simulink model "nnex"  (Simulink 3.00)
settings: Solver=ode4  StartTime=0.0  StopTime=80.0  FixedStep=0.01  RelTol=1e-3
values from neighbouring files (symbols this model uses):
  a = [0 0 0 0 -1.84243174515 0 -13.0175486382 0 -0.783906463276 0 0 0 ... (81 elements, 9x9)]    [abcdkkf.mat]
  b = [0 0 0 0.0409816056965 -1.1184911635 -0.696996430025 -7.90261427727 -0.243253277751 -0.475887299716 0 0 0 ... (72 elements, 9x8)]    [abcdkkf.mat]
  K = [0.205046990931 0.178802882473 0.205046973039 0.231291081498 0.205047227102 0.208989425276 0.205046736869 0.201104538695 0.029790172361 1.88182262784e-07 -0.0297901447303 -1.60551558311e-07 ... (72 elements, 8x9)]    [abcdkkf.mat]
  Kf = [-0.016083954489 -0.0112761944666 -0.0160839192866 -0.020891679309 -0.0160839730143 0.0019082921562 -0.0160839007613 -0.0340761659318 -0.0453569952473 -2.86516704076e-07 0.0453569531782 2.44447604365e-07 ... (24 elements, 8x3)]    [abcdkkf.mat]
undefined symbols (not defined in the file or in its folder): h, Kd, Kp, omega, zeta
libraries: smxl x11, simulink3 x6, neural x2
settings Model: LastModifiedBy=giampiero

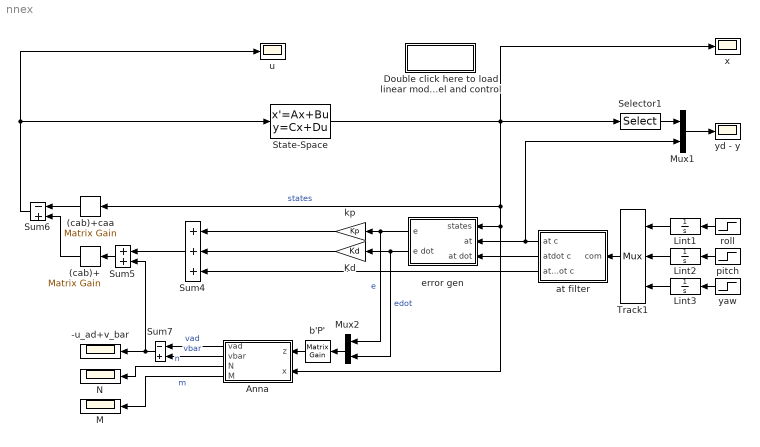
== system nnex ==
  (cab)+ : simulink3/Math/Matrix Gain  Orientation=left  K=Kf
  (cab)+caa : simulink3/Math/Matrix Gain  Orientation=left  K=K
  -u_ad+v_bar : Scope
      settings: TickLabels=off  TimeRange=40  YMin=-250  YMax=50  SaveName=u_nn  DataFormat=Matrix  MaxRows=40000
  Anna : Subsystem  Orientation=left  mask(Adaptive Neural Network){s=[     3    9      6     1       0         0        0], g=[0.1         40     0   40 40           0.01]}
      mask prompts: s "[nno nni nnh act rndN rndM bias]"; g "[Kv   Z_bar   Kz    G   F   lambda]"
      mask help: Continuous Time Adaptive Multilayer MIMO Neural Network.
      mask init:
      | nno=s(1); nni=s(2); nnh=s(3); a=s(4); rndN=s(5);rndM=s(6);
      | bias=s(7); Kv=g(1); Z_bar=g(2);Kz=g(3);G=g(4);F=g(5);lam=g(6);
      mask Help:
      | <html xmlns:o="urn:schemas-microsoft-com:office:office"
      | xmlns:w="urn:schemas-microsoft-com:office:word"
      | xmlns="http://www.w3.org/TR/REC-html40">
      | 
      | <head>
      | <meta http-equiv=Content-Type content="text/html; charset=windows-1252">
      | <meta name=ProgId content=Word.Document>
      | <meta name=Generator content="Microsoft Word 9">
      | <meta name=Originator content="Microsoft Word 9">
      | <link rel=File-List href="./help_files/filelist.xml">
      | <title>Notation and adaptation algorithm are taken from the paper:</title>
      | <!--[if gte mso 9]><xml>
      |  <o:DocumentProperties>
      |   <o:Author>Control Lab</o:Author>
      |   <o:LastAuthor>giampiero</o:LastAuthor>
      |   <o:Revision>14</o:Revision>
      |   <o:TotalTime>134</o:TotalTime>
      |   <o:Created>1999-07-30T18:31:00Z</o:Created>
      |   <o:LastSaved>2000-05-30T23:27:00Z</o:LastSaved>
      |   <o:Pages>1</o:Pages>
      |   <o:Words>234</o:Words>
      |   <o:Characters>1339</o:Characters>
      |   <o:Company>GA TECH</o:Company>
      |   <o:Lines>11</o:Lines>
      |   <o:Paragraphs>2</o:Paragraphs>
      |   <o:CharactersWithSpaces>1644</o:CharactersWithSpaces>
      |   <o:Version>9.2720</o:Version>
      |  </o:DocumentProperties>
      | </xml><![endif]-->
      | <style>
      | <!--
      |  /* Style Definitions */
      | p.MsoNormal, li.MsoNormal, div.MsoNormal
      | 	{mso-style-parent:"";
      | 	margin:0in;
      | 	margin-bottom:.0001pt;
      | 	mso-pagination:widow-orphan;
      | 	font-size:12.0pt;
      | 	font-family:"Times New Roman";
      | 	mso-fareast-font-family:"Times New Roman";}
      | p.MsoBodyText, li.MsoBodyText, div.MsoBodyText
      | 	{margin-top:0in;
      | 	margin-right:3.35in;
      | 	margin-bottom:0in;
      | 	margin-left:0in;
      | 	margin-bottom:.0001pt;
      | 	mso-pagination:widow-orphan;
      | 	font-size:12.0pt;
      | 	font-family:"Times New Roman";
      | 	mso-fareast-font-family:"Times New Roman";}
      | p.MsoBodyText2, li.MsoBodyText2, div.MsoBodyText2
      | 	{margin-top:0in;
      | 	margin-right:2.35in;
      | 	margin-bottom:0in;
      | 	margin-left:0in;
      | 	margin-bottom:.0001pt;
      | 	mso-pagination:widow-orphan;
      | 	font-size:12.0pt;
      | 	font-family:"Times New Roman";
      | 	mso-fareast-font-family:"Times New Roman";}
      | @page Section1
      | 	{size:8.5in 11.0in;
      | 	margin:1.0in 1.25in 1.0in 1.25in;
      | 	mso-header-margin:.5in;
      | 	mso-footer-margin:.5in;
      | 	mso-paper-source:0;}
      | div.Section1
      | 	{page:Section1;}
      |  /* List Definitions */
      | @list l0
      | 	{mso-list-id:387336931;
      | 	mso-list-type:hybrid;
      | 	mso-list-template-ids:1661509918 67698705 67698713 67698715 67698703 67698713 67698715 67698703 67698713 67698715;}
      | @list l0:level1
      | 	{mso-level-text:"%1\)";
      | 	mso-level-tab-stop:.5in;
      | 	mso-level-number-position:left;
      | 	text-indent:-.25in;}
      | @list l1
      | 	{mso-list-id:1390807613;
      | 	mso-list-type:hybrid;
      | 	mso-list-template-ids:210782786 67698705 67698713 67698715 67698703 67698713 67698715 67698703 67698713 67698715;}
      | @list l1:level1
      | 	{mso-level-text:"%1\)";
      | 	mso-level-tab-stop:.5in;
      | 	mso-level-number-position:left;
      | 	text-indent:-.25in;}
      | @list l2
      | 	{mso-list-id:1468430361;
      | 	mso-list-type:hybrid;
      | 	mso-list-template-ids:-783395272 67698705 67698713 67698715 67698703 67698713 67698715 67698703 67698713 67698715;}
      | @list l2:level1
      | 	{mso-level-text:"%1\)";
      | 	mso-level-tab-stop:.5in;
      | 	mso-level-number-position:left;
      | 	text-indent:-.25in;}
      | @list l3
      | 	{mso-list-id:2055232913;
      | 	mso-list-type:hybrid;
      | 	mso-list-template-ids:-1797358054 67698705 67698713 67698715 67698703 67698713 67698715 67698703 67698713 67698715;}
      | @list l3:level1
      | 	{mso-level-text:"%1\)";
      | 	mso-level-tab-stop:.5in;
      | 	mso-level-number-position:left;
      | 	text-indent:-.25in;}
      | ol
      | 	{margin-bottom:0in;}
      | ul
      | 	{margin-bottom:0in;}
      | -->
      | </style>
      | </head>
      | 
      | <body lang=EN-US style='tab-interval:.5in'>
      | 
      | <div class=Section1>
      | 
      | <p class=MsoBodyText2 style='margin-right:-1.8pt'>The block implements a
      | continuous time adaptive multilayer MIMO sigmoidal neural network, this is a
      | simulink based version that uses the Transposition and Multiplication blocks from the Smxl Library, therefore you must have that library in your Matlab path in order to use this block.</p>
      | 
      | <p class=MsoNormal style='margin-right:-1.8pt'><![if !supportEmptyParas]>&nbsp;<![endif]><o:p></o:p></p>
      | 
      | <p class=MsoNormal style='margin-right:-1.8pt'>Notation and adaptation
      | algorithm are taken from the paper:</p>
      | 
      | <p class=MsoBodyText style='margin-right:-1.8pt'>Neural Network Based Adaptive
      | Control of a Thrust Vectored Fan, Nardi, Rysdik, Calise, AIAA 1999-3996, where
      | the used neural network has the equations shown below:</p>
      | 
      | <p class=MsoBodyText style='margin-right:-1.8pt'><![if !supportEmptyParas]>&nbsp;<![endif]><o:p></o:p></p>
      | 
      | <p class=MsoBodyText style='margin-right:-1.8pt;tab-stops:27.0pt'>N<sub>dot<span
      | style='mso-tab-count:1'>    </span></sub>= -G[x<sub>bar</sub><span
      | style='font-family:Symbol;mso-ascii-font-family:"Times New Roman";mso-hansi-font-family:
      | "Times New Roman";mso-char-type:symbol;mso-symbol-font-family:Symbol'><span
      | style='mso-char-type:symbol;mso-symbol-font-family:Symbol'>z</span></span>M<sup>T</sup><span
      | style='font-family:Symbol;mso-ascii-font-family:"Times New Roman";mso-hansi-font-family:
      | "Times New Roman";mso-char-type:symbol;mso-symbol-font-family:Symbol'><span
      | style='mso-char-type:symbol;mso-symbol-font-family:Symbol'>s</span></span>’(N<sup>T</sup>x<sub>bar</sub>)
      | + <span style='font-family:Symbol;mso-ascii-font-family:"Times New Roman";
      | mso-hansi-font-family:"Times New Roman";mso-char-type:symbol;mso-symbol-font-family:
      | Symbol'><span style='mso-char-type:symbol;mso-symbol-font-family:Symbol'>l</span></span><span
      | style='font-family:Symbol;mso-ascii-font-family:"Times New Roman";mso-hansi-font-family:
      | "Times New Roman";mso-char-type:symbol;mso-symbol-font-family:Symbol'><span
      | style='mso-char-type:symbol;mso-symbol-font-family:Symbol'>ï</span></span><span
      | style='font-family:Symbol;mso-ascii-font-family:"Times New Roman";mso-hansi-font-family:
      | "Times New Roman";mso-char-type:symbol;mso-symbol-font-family:Symbol'><span
      | style='mso-char-type:symbol;mso-symbol-font-family:Symbol'>z</span></span><span
      | style='font-family:Symbol;mso-ascii-font-family:"Times New Roman";mso-hansi-font-family:
      | "Times New Roman";mso-char-type:symbol;mso-symbol-font-family:Symbol'><span
      | style='mso-char-type:symbol;mso-symbol-font-family:Symbol'>ï</span></span>N]</p>
      | 
      | <p class=MsoBodyText style='margin-right:-1.8pt;tab-stops:27.0pt'>N<sub>dot<span
      | style='mso-tab-count:1'>    </span></sub>= -F[(<span style='font-family:Symbol;
      | mso-ascii-font-family:"Times New Roman";mso-hansi-font-family:"Times New Roman";
      | mso-char-type:symbol;mso-symbol-font-family:Symbol'><span style='mso-char-type:
      | symbol;mso-symbol-font-family:Symbol'>s</span></span>(N<sup>T</sup>x<sub>bar</sub>)-<span
      | style='font-family:Symbol;mso-ascii-font-family:"Times New Roman";mso-hansi-font-family:
      | "Times New Roman";mso-char-type:symbol;mso-symbol-font-family:Symbol'><span
      | style='mso-char-type:symbol;mso-symbol-font-family:Symbol'>s</span></span>’(N<sup>T</sup>x<sub>bar</sub>)N<sup>T</sup>x<sub>bar</sub>)<span
      | style='font-family:Symbol;mso-ascii-font-family:"Times New Roman";mso-hansi-font-family:
      | "Times New Roman";mso-char-type:symbol;mso-symbol-font-family:Symbol'><span
      | style='mso-char-type:symbol;mso-symbol-font-family:Symbol'>z</span></span> + <span
      | style='font-family:Symbol;mso-ascii-font-family:"Times New Roman";mso-hansi-font-family:
      | "Times New Roman";mso-char-type:symbol;mso-symbol-font-family:Symbol'><span
      | style='mso-char-type:symbol;mso-symbol-font-family:Symbol'>l</span></span><span
      | style='font-family:Symbol;mso-ascii-font-family:"Times New Roman";mso-hansi-font-family:
      | "Times New Roman";mso-char-type:symbol;mso-symbol-font-family:Symbol'><span
      | style='mso-char-type:symbol;mso-symbol-font-family:Symbol'>ï</span></span><span
      | style='font-family:Symbol;mso-ascii-font-family:"Times New Roman";mso-hansi-font-family:
      | "Times New Roman";mso-char-type:symbol;mso-symbol-font-family:Symbol'><span
      | style='mso-char-type:symbol;mso-symbol-font-family:Symbol'>z</span></span><span
      | style='font-family:Symbol;mso-ascii-font-family:"Times New Roman";mso-hansi-font-family:
      | "Times New Roman";mso-char-type:symbol;mso-symbol-font-family:Symbol'><span
      | style='mso-char-type:symbol;mso-symbol-font-family:Symbol'>ï</span></span>M]</p>
      | 
      | <p class=MsoBodyText style='margin-right:-1.8pt;tab-stops:27.0pt'>v<sub>ad<span
      | style='mso-tab-count:1'>       </span></sub>= <span style="mso-spacerun:
      | yes"> </span>M<sup>T</sup><span style='font-family:Symbol;mso-ascii-font-family:
      | "Times New Roman";mso-hansi-font-family:"Times New Roman";mso-char-type:symbol;
      | mso-symbol-font-family:Symbol'><span style='mso-char-type:symbol;mso-symbol-font-family:
      | Symbol'>s</span></span>(N<sup>T</sup>x<sub>bar</sub>)</p>
      | 
      | <p class=MsoBodyText style='margin-right:-1.8pt;tab-stops:27.0pt'>v<sub>bar<span
      | style='mso-tab-count:1'>      </span></sub>= <span style="mso-spacerun:
      | yes"> </span>K<sub>v</sub> (<span style='font-family:Symbol;mso-ascii-font-family:
      | "Times New Roman";mso-hansi-font-family:"Times New Roman";mso-char-type:symbol;
      | mso-symbol-font-family:Symbol'><span style='mso-char-type:symbol;mso-symbol-font-family:
      | Symbol'>ï</span></span>Z<span style='font-family:Symbol;mso-ascii-font-family:
      | "Times New Roman";mso-hansi-font-family:"Times New Roman";mso-char-type:symbol;
      | mso-symbol-font-family:Symbol'><span style='mso-char-type:symbol;mso-symbol-font-family:
      | Symbol'>ï</span></span><sub>F</sub> + Z<sub>bar</sub>)<span style='font-family:
      | Symbol;mso-ascii-font-family:"Times New Roman";mso-hansi-font-family:"Times New Roman";
      | mso-char-type:symbol;mso-symbol-font-family:Symbol'><span style='mso-char-type:
      | symbol;mso-symbol-font-family:Symbol'>z</span></span><sup>T</sup> + K<sub>z</sub><span
      | style='font-family:Symbol;mso-ascii-font-family:"Times New Roman";mso-hansi-font-family:
      | "Times New Roman";mso-char-type:symbol;mso-symbol-font-family:Symbol'><span
      | style='mso-char-type:symbol;mso-symbol-font-family:Symbol'>z</span></span><sup>T</sup></p>
      | 
      | <p class=MsoBodyText style='margin-right:-1.8pt'><![if !supportEmptyParas]>&nbsp;<![endif]><o:p></o:p></p>
      | 
      | <p class=MsoNormal style='margin-right:-1.8pt'>The <u>Inputs</u> are:</p>
      | 
      | <p class=MsoNormal style='margin-top:0in;margin-right:-1.8pt;margin-bottom:
      | 0in;margin-left:.5in;margin-bottom:.0001pt;text-indent:-.25in;mso-list:l2 level1 lfo2;
      | tab-stops:list .5in'><![if !supportLists]>1)<span style='font:7.0pt "Times New Roman"'>&nbsp;&nbsp;&nbsp;&nbsp;&nbsp;
      | </span><![endif]>error vector <span style='font-family:Symbol;mso-ascii-font-family:
      | "Times New Roman";mso-hansi-font-family:"Times New Roman";mso-char-type:symbol;
      | mso-symbol-font-family:Symbol'><span style='mso-char-type:symbol;mso-symbol-font-family:
      | Symbol'>z</span></span> (<span style='font-family:Symbol;mso-ascii-font-family:
      | "Times New Roman";mso-hansi-font-family:"Times New Roman";mso-char-type:symbol;
      | mso-symbol-font-family:Symbol'><span style='mso-char-type:symbol;mso-symbol-font-family:
      | Symbol'>z</span></span>=ePb).</p>
      | 
      | <p class=MsoNormal style='margin-top:0in;margin-right:-1.8pt;margin-bottom:
      | 0in;margin-left:.5in;margin-bottom:.0001pt;text-indent:-.25in;mso-list:l2 level1 lfo2;
      | tab-stops:list .5in'><![if !supportLists]>2)<span style='font:7.0pt "Times New Roman"'>&nbsp;&nbsp;&nbsp;&nbsp;&nbsp;
      | </span><![endif]>net input vector x<sub>bar</sub> (x<sub>bar</sub>=[x,u]).</p>
      | 
      | <p class=MsoNormal style='margin-right:-1.8pt'><![if !supportEmptyParas]>&nbsp;<![endif]><o:p></o:p></p>
      | 
      | <p class=MsoNormal style='margin-right:-1.8pt'>The <u>States</u> are all N and
      | M entries.</p>
      | 
      | <p class=MsoNormal style='margin-right:-1.8pt'><![if !supportEmptyParas]>&nbsp;<![endif]><o:p></o:p></p>
      | 
      | <p class=MsoNormal style='margin-right:-1.8pt;text-align:justify'>The <u>Outputs</u>
      | are:</p>
      | 
      | <p class=MsoNormal style='margin-top:0in;margin-right:-1.8pt;margin-bottom:
      | 0in;margin-left:.5in;margin-bottom:.0001pt;text-indent:-.25in;mso-list:l1 level1 lfo4;
      | tab-stops:list .5in'><![if !supportLists]>1)<span style='font:7.0pt "Times New Roman"'>&nbsp;&nbsp;&nbsp;&nbsp;&nbsp;
      | </span><![endif]>v<sub>ad</sub> (adaptive contribution).</p>
      | 
      | <p class=MsoNormal style='margin-top:0in;margin-right:-1.8pt;margin-bottom:
      | 0in;margin-left:.5in;margin-bottom:.0001pt;text-indent:-.25in;mso-list:l1 level1 lfo4;
      | tab-stops:list .5in'><![if !supportLists]>2)<span style='font:7.0pt "Times New Roman"'>&nbsp;&nbsp;&nbsp;&nbsp;&nbsp;
      | </span><![endif]>v<sub>bar</sub> ( robustifying contribution).</p>
      | 
      | <p class=MsoNormal style='margin-top:0in;margin-right:-1.8pt;margin-bottom:
      | 0in;margin-left:.5in;margin-bottom:.0001pt;text-indent:-.25in;mso-list:l1 level1 lfo4;
      | tab-stops:list .5in'><![if !supportLists]>3)<span style='font:7.0pt "Times New Roman"'>&nbsp;&nbsp;&nbsp;&nbsp;&nbsp;
      | </span><![endif]>N entries taken columnwise.</p>
      | 
      | <p class=MsoNormal style='margin-top:0in;margin-right:-1.8pt;margin-bottom:
      | 0in;margin-left:.5in;margin-bottom:.0001pt;text-indent:-.25in;mso-list:l1 level1 lfo4;
      | tab-stops:list .5in'><![if !supportLists]>4)<span style='font:7.0pt "Times New Roman"'>&nbsp;&nbsp;&nbsp;&nbsp;&nbsp;
      | </span><![endif]>M entries taken columnwise.</p>
      | 
      | <p class=MsoNormal style='margin-right:-1.8pt'><![if !supportEmptyParas]>&nbsp;<![endif]><o:p></o:p></p>
      | 
      | <p class=MsoNormal style='margin-right:-1.8pt'>The <u>first</u> parameter must
      | be a vector containing:</p>
      | 
      | <p class=MsoNormal style='margin-top:0in;margin-right:-1.8pt;margin-bottom:
      | 0in;margin-left:.5in;margin-bottom:.0001pt;text-indent:-.25in;mso-list:l0 level1 lfo6;
      | tab-stops:list .5in'><![if !supportLists]>1)<span style='font:7.0pt "Times New Roman"'>&nbsp;&nbsp;&nbsp;&nbsp;&nbsp;
      | </span><![endif]>nno = number of network output = size of the error.</p>
      | 
      | <p class=MsoNormal style='margin-top:0in;margin-right:-1.8pt;margin-bottom:
      | 0in;margin-left:.5in;margin-bottom:.0001pt;text-indent:-.25in;mso-list:l0 level1 lfo6;
      | tab-stops:list .5in'><![if !supportLists]>2)<span style='font:7.0pt "Times New Roman"'>&nbsp;&nbsp;&nbsp;&nbsp;&nbsp;
      | </span><![endif]>nni = number of network inputs = plant states.</p>
      | 
      | <p class=MsoNormal style='margin-top:0in;margin-right:-1.8pt;margin-bottom:
      | 0in;margin-left:.5in;margin-bottom:.0001pt;text-indent:-.25in;mso-list:l0 level1 lfo6;
      | tab-stops:list .5in'><![if !supportLists]>3)<span style='font:7.0pt "Times New Roman"'>&nbsp;&nbsp;&nbsp;&nbsp;&nbsp;
      | </span><![endif]>nnh = number of hidden layer neurons.</p>
      | 
      | <p class=MsoNormal style='margin-top:0in;margin-right:-1.8pt;margin-bottom:
      | 0in;margin-left:.5in;margin-bottom:.0001pt;text-indent:-.25in;mso-list:l0 level1 lfo6;
      | tab-stops:list .5in'><![if !supportLists]>4)<span style='font:7.0pt "Times New Roman"'>&nbsp;&nbsp;&nbsp;&nbsp;&nbsp;
      | </span><![endif]>act = sigmoid activation potential.</p>
      | 
      | <p class=MsoNormal style='margin-top:0in;margin-right:-1.8pt;margin-bottom:
      | 0in;margin-left:.5in;margin-bottom:.0001pt;text-indent:-.25in;mso-list:l0 level1 lfo6;
      | tab-stops:list .5in'><![if !supportLists]>5)<span style='font:7.0pt "Times New Roman"'>&nbsp;&nbsp;&nbsp;&nbsp;&nbsp;
      | </span><![endif]>rndN = multiplies random initial weights N.</p>
      | 
      | <p class=MsoNormal style='margin-top:0in;margin-right:-1.8pt;margin-bottom:
      | 0in;margin-left:.5in;margin-bottom:.0001pt;text-indent:-.25in;mso-list:l0 level1 lfo6;
      | tab-stops:list .5in'><![if !supportLists]>6)<span style='font:7.0pt "Times New Roman"'>&nbsp;&nbsp;&nbsp;&nbsp;&nbsp;
      | </span><![endif]>rndM = multiplies random initial weights M.</p>
      | 
      | <p class=MsoNormal style='margin-top:0in;margin-right:-1.8pt;margin-bottom:
      | 0in;margin-left:.5in;margin-bottom:.0001pt;text-indent:-.25in;mso-list:l0 level1 lfo6;
      | tab-stops:list .5in'><![if !supportLists]>7)<span style='font:7.0pt "Times New Roman"'>&nbsp;&nbsp;&nbsp;&nbsp;&nbsp;
      | </span><![endif]>bias = put 1 if you want it, 0 otherwise.</p>
      | 
      | <p class=MsoNormal style='margin-right:-1.8pt'><![if !supportEmptyParas]>&nbsp;<![endif]><o:p></o:p></p>
      | 
      | <p class=MsoBodyText style='margin-right:-1.8pt'>The <u>second</u> parameter
      | must be a vector containing:</p>
      | 
      | <p class=MsoNormal style='margin-top:0in;margin-right:-1.8pt;margin-bottom:
      | 0in;margin-left:.5in;margin-bottom:.0001pt;text-indent:-.25in;mso-list:l3 level1 lfo8;
      | tab-stops:list .5in'><![if !supportLists]>1)<span style='font:7.0pt "Times New Roman"'>&nbsp;&nbsp;&nbsp;&nbsp;&nbsp;
      | </span><![endif]>K<sub>v</sub> = multiplies first term of v<sub>bar</sub>.</p>
      | 
      | <p class=MsoNormal style='margin-top:0in;margin-right:-1.8pt;margin-bottom:
      | 0in;margin-left:.5in;margin-bottom:.0001pt;text-indent:-.25in;mso-list:l3 level1 lfo8;
      | tab-stops:list .5in'><![if !supportLists]>2)<span style='font:7.0pt "Times New Roman"'>&nbsp;&nbsp;&nbsp;&nbsp;&nbsp;
      | </span><![endif]>Z<sub>bar</sub> = maximum expected <span style='font-family:
      | Symbol;mso-ascii-font-family:"Times New Roman";mso-hansi-font-family:"Times New Roman";
      | mso-char-type:symbol;mso-symbol-font-family:Symbol'><span style='mso-char-type:
      | symbol;mso-symbol-font-family:Symbol'>ï</span></span>Z<span style='font-family:
      | Symbol;mso-ascii-font-family:"Times New Roman";mso-hansi-font-family:"Times New Roman";
      | mso-char-type:symbol;mso-symbol-font-family:Symbol'><span style='mso-char-type:
      | symbol;mso-symbol-font-family:Symbol'>ï</span></span><sub>F</sub> value (see v<sub>bar</sub>).</p>
      | 
      | <p class=MsoNormal style='margin-top:0in;margin-right:-1.8pt;margin-bottom:
      | 0in;margin-left:.5in;margin-bottom:.0001pt;text-indent:-.25in;mso-list:l3 level1 lfo8;
      | tab-stops:list .5in'><![if !supportLists]>3)<span style='font:7.0pt "Times New Roman"'>&nbsp;&nbsp;&nbsp;&nbsp;&nbsp;
      | </span><![endif]>K<sub>z</sub> = multiplies second term of v<sub>bar</sub>.</p>
      | 
      | <p class=MsoNormal style='margin-top:0in;margin-right:-1.8pt;margin-bottom:
      | 0in;margin-left:.5in;margin-bottom:.0001pt;text-indent:-.25in;mso-list:l3 level1 lfo8;
      | tab-stops:list .5in'><![if !supportLists]>4)<span style='font:7.0pt "Times New Roman"'>&nbsp;&nbsp;&nbsp;&nbsp;&nbsp;
      | </span><![endif]>G = learning rate of N (input layer).</p>
      | 
      | <p class=MsoNormal style='margin-top:0in;margin-right:-1.8pt;margin-bottom:
      | 0in;margin-left:.5in;margin-bottom:.0001pt;text-indent:-.25in;mso-list:l3 level1 lfo8;
      | tab-stops:list .5in'><![if !supportLists]>5)<span style='font:7.0pt "Times New Roman"'>&nbsp;&nbsp;&nbsp;&nbsp;&nbsp;
      | </span><![endif]>F = learning rate of M (output layer).</p>
      | 
      | <p class=MsoNormal style='margin-top:0in;margin-right:-1.8pt;margin-bottom:
      | 0in;margin-left:.5in;margin-bottom:.0001pt;text-indent:-.25in;mso-list:l3 level1 lfo8;
      | tab-stops:list .5in'><![if !supportLists]>6)<span style='font:7.0pt "Times New Roman"'>&nbsp;&nbsp;&nbsp;&nbsp;&nbsp;
      | </span><![endif]>lambda (e modification) = coefficient multiplying <span
      | style='font-family:Symbol;mso-ascii-font-family:"Times New Roman";mso-hansi-font-family:
      | "Times New Roman";mso-char-type:symbol;mso-symbol-font-family:Symbol'><span
      | style='mso-char-type:symbol;mso-symbol-font-family:Symbol'>z</span></span> in
      | the adaptation laws.</p>
      | 
      | <p class=MsoNormal style='margin-right:-1.8pt'><![if !supportEmptyParas]>&nbsp;<![endif]><o:p></o:p></p>
      | 
      | <p class=MsoNormal style='margin-right:-1.8pt'>Developed by Giampiero Campa in
      | Aug99, email: gcampa@dsea.unipi.it</p>
      | 
      | </div>
      | 
      | </body>
      | 
      | </html>
      mask Display: plot(0,0,100,100,[80,20],[90,70],[80,20],[50,50],[80,20],[10,30],[80,20],[50,30],[80,21],[90,30],[80,20],[10,50],[80,21],[91,50],[80,20],[50,70],[80,20],[10,70])
  "Double click here to load linear model and control " : Subsystem
      settings: OpenFcn=h=0.3;zeta=1;omega=3;Kp=omega^2;Kd=2*omega;load abcdkkf
      mask Display: disp('Load Model')
  Kd : Gain  Orientation=left  Gain=Kd  SaturateOnIntegerOverflow=on
  Lint1 : Integrator  Orientation=left  ExternalReset=none  InitialConditionSource=internal  InitialCondition=0  LimitOutput=on  UpperSaturationLimit=h  LowerSaturationLimit=-h  ShowSaturationPort=off  ShowStatePort=off  AbsoluteTolerance=auto
  Lint2 : Integrator  Orientation=left  ExternalReset=none  InitialConditionSource=internal  InitialCondition=0  LimitOutput=on  UpperSaturationLimit=h  LowerSaturationLimit=-h  ShowSaturationPort=off  ShowStatePort=off  AbsoluteTolerance=auto
  Lint3 : Integrator  Orientation=left  ExternalReset=none  InitialConditionSource=internal  InitialCondition=0  LimitOutput=on  UpperSaturationLimit=h  LowerSaturationLimit=-h  ShowSaturationPort=off  ShowStatePort=off  AbsoluteTolerance=auto
  M : Scope
      settings: TickLabels=off  TimeRange=40  YMin=-25  YMax=55  SaveName=weight_M  DataFormat=Matrix  MaxRows=40000
  Mux1 : Mux  Inputs=2
  Mux2 : Mux  Orientation=left  Inputs=2
  N : Scope
      settings: TickLabels=off  TimeRange=40  YMin=-25  YMax=55  SaveName=weight_N  DataFormat=Matrix  MaxRows=40000
  Selector1 : Selector  Elements=[1 2 3]  InputPortWidth=9
  State-Space : StateSpace  A=a  B=b  C=eye(9)  D=zeros(9,8)  X0=0
  Sum4 : Sum  Orientation=left  Inputs=+++  SaturateOnIntegerOverflow=on
  Sum5 : Sum  Orientation=left  Inputs=++  SaturateOnIntegerOverflow=on
  Sum6 : Sum  Orientation=left  Inputs=-+  SaturateOnIntegerOverflow=on
  Sum7 : Sum  Orientation=left  Inputs=-+  SaturateOnIntegerOverflow=on
  Track1 : Mux  Orientation=left  Inputs=3
      settings: DisplayOption=none
  at filter : Subsystem  Orientation=left
  b'P' : simulink3/Math/Matrix Gain  Orientation=left  K=[eye(3)*1/(2*Kp) eye(3)*(Kp + 1)/(2*Kp*Kd)]
  error gen : Subsystem  Orientation=left
  kp : Gain  Orientation=left  Gain=Kp  SaturateOnIntegerOverflow=on
  pitch : Step  Orientation=left  Time=30  Before=0  After=0.1  SampleTime=.01
  roll : Step  Orientation=left  Time=40  Before=0  After=0.1  SampleTime=.01
  u : Scope
      settings: TickLabels=off  TimeRange=40  YMin=-0.7  YMax=0.5  SaveName=u  DataFormat=Matrix  MaxRows=40000
  x : Scope
      settings: TickLabels=off  TimeRange=40  YMin=-0.25  YMax=1.75  SaveName=x  DataFormat=Matrix  MaxRows=40000
  yaw : Step  Orientation=left  Time=20  Before=0  After=0.1  SampleTime=.01
  yd - y : Scope
      settings: TickLabels=off  TimeRange=10  YMin=-0.05  YMax=0.35  SaveName=th  DataFormat=Matrix  MaxRows=40000
  wires:
  Sum4/1 -> Sum5/1
  Kd/1 -> Sum4/2
  kp/1 -> Sum4/1
  error gen/1(e) -> kp/1, Mux2/1  "e"
  error gen/2(e dot) -> Kd/1, Mux2/2  "edot"
  at filter/2(atdot c) -> error gen/3(at dot)
  at filter/3(atddot c) -> Sum4/3
  at filter/1(at c) -> error gen/2(at), Mux1/2
  Track1/1 -> at filter/1(com)
  roll/1 -> Lint1/1
  pitch/1 -> Lint2/1
  yaw/1 -> Lint3/1
  Lint1/1 -> Track1/1
  Lint2/1 -> Track1/2
  Lint3/1 -> Track1/3
  Anna/2(vbar) -> Sum7/2  "vbar"
  Anna/1(vad) -> Sum7/1  "vad"
  Mux2/1 -> b'P'/1
  b'P'/1 -> Anna/1(z)
  (cab)+caa/1 -> Sum6/1
  (cab)+/1 -> Sum6/2
  Sum5/1 -> (cab)+/1
  Sum7/1 -> -u_ad+v_bar/1, Sum5/2
  Anna/3(N) -> N/1  "n"
  Anna/4(M) -> M/1  "m"
  Sum6/1 -> u/1, State-Space/1
  State-Space/1 -> x/1, (cab)+caa/1, error gen/1(states), Anna/2(x), Selector1/1  "states"
  Mux1/1 -> yd - y/1
  Selector1/1 -> Mux1/1

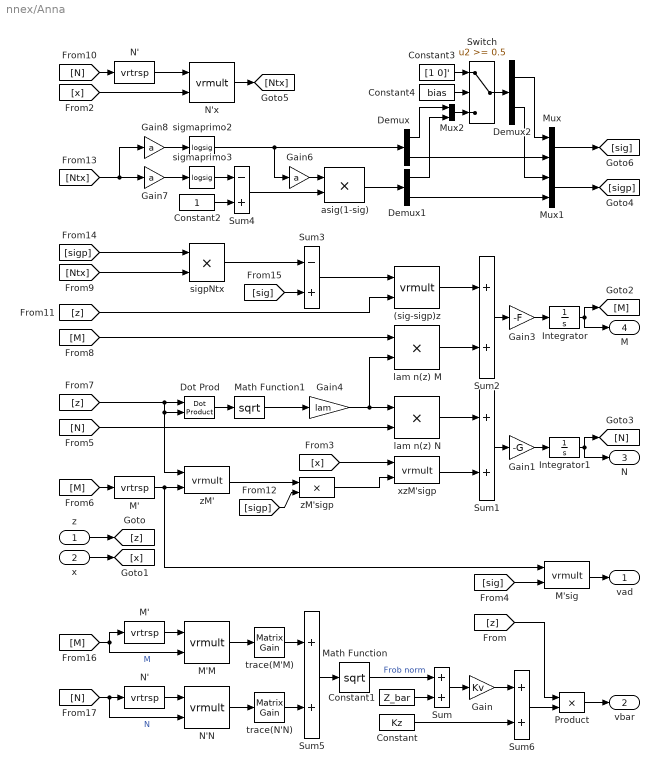
== system nnex/Anna ==
  z : Inport  Port=1  PortWidth=-1  SampleTime=-1  DataType=auto
      settings: SignalType=auto
  x : Inport  Port=2  PortWidth=-1  SampleTime=-1  DataType=auto
      settings: SignalType=auto
  (sig-sigp)z : smxl/Real Matrices/vrmult  dims=[nnh 1 nno]
  Constant : Constant  Value=Kz
  Constant1 : Constant  Value=Z_bar
  Constant2 : Constant  Value=1
  Constant3 : Constant  Value=[1 0]'
  Constant4 : Constant  Value=bias
  Demux : Demux  Outputs=[1 nnh-1]
  Demux1 : Demux  Outputs=[1 nnh-1]
  Demux2 : Demux  Outputs=[1 1]
  Dot Prod : simulink3/Math/Dot Product
  Gain : Gain  Gain=Kv  SaturateOnIntegerOverflow=on
  Gain1 : Gain  Gain=-G  SaturateOnIntegerOverflow=on
  Gain3 : Gain  Gain=-F  SaturateOnIntegerOverflow=on
  Gain4 : Gain  Gain=lam  SaturateOnIntegerOverflow=on
  Gain6 : Gain  Gain=a  SaturateOnIntegerOverflow=on
  Gain7 : Gain  Gain=a  SaturateOnIntegerOverflow=on
  Gain8 : Gain  Gain=a  SaturateOnIntegerOverflow=on
  Integrator : Integrator  ExternalReset=none  InitialConditionSource=internal  InitialCondition=rndM*rand(nnh*nno,1)  LimitOutput=off  UpperSaturationLimit=inf  LowerSaturationLimit=-inf  ShowSaturationPort=off  ShowStatePort=off  AbsoluteTolerance=auto
  Integrator1 : Integrator  ExternalReset=none  InitialConditionSource=internal  InitialCondition=rndN*rand(nni*nnh,1)  LimitOutput=off  UpperSaturationLimit=inf  LowerSaturationLimit=-inf  ShowSaturationPort=off  ShowStatePort=off  AbsoluteTolerance=auto
  M' : smxl/Real Matrices/vrtrsp  dims=[nnh nno]
  "M' " : smxl/Real Matrices/vrtrsp  dims=[nnh nno]
  M'M : smxl/Real Matrices/vrmult  dims=[nno nnh nno]
  M'sig : smxl/Real Matrices/vrmult  dims=[nno nnh 1]
  Math Function : Math  Operator=sqrt  OutputSignalType=real
  Math Function1 : Math  Operator=sqrt  OutputSignalType=real
  Mux : Mux  Inputs=[1 nnh-1]
  Mux1 : Mux  Inputs=[1 nnh-1]
  Mux2 : Mux  Inputs=[1 1]
  N' : smxl/Real Matrices/vrtrsp  dims=[nni nnh]
  "N' " : smxl/Real Matrices/vrtrsp  dims=[nni nnh]
  N'N : smxl/Real Matrices/vrmult  dims=[nnh nni nnh]
  N'x : smxl/Real Matrices/vrmult  dims=[nnh nni 1]
  Product : Product  Inputs=2  SaturateOnIntegerOverflow=on
  Sum{,1..2,5..6} (5 alike) : Sum  Inputs=++  SaturateOnIntegerOverflow=on
  Sum3 : Sum  Inputs=-+  SaturateOnIntegerOverflow=on
  Sum4 : Sum  Inputs=-+  SaturateOnIntegerOverflow=on
  Switch : Switch  Threshold=0.5
  asig(1-sig) : Product  Inputs=2  SaturateOnIntegerOverflow=on
  lam n(z) M : Product  Inputs=2  SaturateOnIntegerOverflow=on
  lam n(z) N : Product  Inputs=2  SaturateOnIntegerOverflow=on
  sigmaprimo2 : neural/Transfer Functions/logsig
  sigmaprimo3 : neural/Transfer Functions/logsig
  sigpNtx : Product  Inputs=2  SaturateOnIntegerOverflow=on
  trace(M'M) : simulink3/Math/Matrix Gain  K=reshape(eye(nno),1,nno^2)
  trace(N'N) : simulink3/Math/Matrix Gain  K=reshape(eye(nnh),1,nnh^2)
  xzM'sigp : smxl/Real Matrices/vrmult  dims=[nni 1 nnh]
  zM' : smxl/Real Matrices/vrmult  dims=[1 nno nnh]
  zM'sigp : Product  Inputs=2  SaturateOnIntegerOverflow=on
  vad : Outport  Port=1
  vbar : Outport  Port=2
  N : Outport  Port=3
  M : Outport  Port=4
  wires:
  N'x/1 -> [Ntx]
  Demux1/1 -> Mux2/2
  Demux/1 -> Mux2/1
  Demux2/1 -> Mux/1
  Demux2/2 -> Mux1/1
  Switch/1 -> Demux2/1
  Mux2/1 -> Switch/3
  Constant4/1 -> Switch/2
  Constant3/1 -> Switch/1
  sigmaprimo2/1 -> Demux/1, Gain6/1
  Sum4/1 -> asig(1-sig)/2
  sigmaprimo3/1 -> Sum4/1
  [Ntx] -> Gain8/1, Gain7/1
  Gain8/1 -> sigmaprimo2/1
  Gain7/1 -> sigmaprimo3/1
  Constant2/1 -> Sum4/2
  asig(1-sig)/1 -> Demux1/1
  Gain6/1 -> asig(1-sig)/1
  Demux1/2 -> Mux1/2
  Demux/2 -> Mux/2
  Mux1/1 -> [sigp]
  Mux/1 -> [sig]
  [x] -> N'x/2
  N'/1 -> N'x/1
  [N] -> N'/1
  N'N/1 -> trace(N'N)/1
  M'M/1 -> trace(M'M)/1
  "M' "/1 -> M'M/1
  [M] -> M'M/2, "M' "/1  "M"
  trace(M'M)/1 -> Sum5/1
  Integrator/1 -> M/1, [M]
  Gain3/1 -> Integrator/1
  z/1 -> [z]
  x/1 -> [x]
  M'/1 -> M'sig/1, zM'/2
  [M] -> M'/1
  [sigp] -> zM'sigp/2
  zM'/1 -> zM'sigp/1
  zM'sigp/1 -> xzM'sigp/2
  [x] -> xzM'sigp/1
  xzM'sigp/1 -> Sum1/2
  lam n(z) N/1 -> Sum1/1
  Sum1/1 -> Gain1/1
  Math Function1/1 -> Gain4/1
  Dot Prod/1 -> Math Function1/1
  [z] -> (sig-sigp)z/2
  sigpNtx/1 -> Sum3/1
  [sig] -> Sum3/2
  Sum3/1 -> (sig-sigp)z/1
  [Ntx] -> sigpNtx/2
  [sigp] -> sigpNtx/1
  Product/1 -> vbar/1
  Sum6/1 -> Product/2
  [z] -> Product/1
  Constant/1 -> Sum6/2
  Gain/1 -> Sum6/1
  Sum/1 -> Gain/1
  [N] -> N'N/2, "N' "/1  "N"
  "N' "/1 -> N'N/1
  Sum5/1 -> Math Function/1
  trace(N'N)/1 -> Sum5/2
  Math Function/1 -> Sum/1  "Frob norm"
  Constant1/1 -> Sum/2
  [sig] -> M'sig/2
  M'sig/1 -> vad/1
  [M] -> lam n(z) M/1
  [z] -> Dot Prod/2, zM'/1, Dot Prod/1
  Gain4/1 -> lam n(z) M/2, lam n(z) N/1
  lam n(z) M/1 -> Sum2/2
  (sig-sigp)z/1 -> Sum2/1
  [N] -> lam n(z) N/2
  Sum2/1 -> Gain3/1
  Integrator1/1 -> N/1, [N]
  Gain1/1 -> Integrator1/1

== system nnex/Double click here to load linear model and control  ==

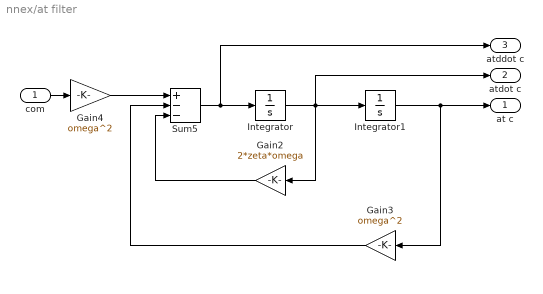
== system nnex/at filter ==
  com : Inport  Port=1  PortWidth=-1  SampleTime=-1  DataType=auto
      settings: SignalType=auto
  Gain2 : Gain  Orientation=left  Gain=2*zeta*omega  SaturateOnIntegerOverflow=on
  Gain3 : Gain  Orientation=left  Gain=omega^2  SaturateOnIntegerOverflow=on
  Gain4 : Gain  Gain=omega^2  SaturateOnIntegerOverflow=on
  Integrator : Integrator  ExternalReset=none  InitialConditionSource=internal  InitialCondition=[0 0 0]'  LimitOutput=off  UpperSaturationLimit=inf  LowerSaturationLimit=-inf  ShowSaturationPort=off  ShowStatePort=off  AbsoluteTolerance=auto
  Integrator1 : Integrator  ExternalReset=none  InitialConditionSource=internal  InitialCondition=[0 0 0]'  LimitOutput=off  UpperSaturationLimit=inf  LowerSaturationLimit=-inf  ShowSaturationPort=off  ShowStatePort=off  AbsoluteTolerance=auto
  Sum5 : Sum  Inputs=+--  SaturateOnIntegerOverflow=on
  at c : Outport  Port=1  InitialOutput=0
  atdot c : Outport  Port=2  InitialOutput=0
  atddot c : Outport  Port=3  InitialOutput=0
  wires:
  com/1 -> Gain4/1
  Gain4/1 -> Sum5/1
  Sum5/1 -> atddot c/1, Integrator/1
  Integrator/1 -> atdot c/1, Gain2/1, Integrator1/1
  Gain2/1 -> Sum5/3
  Gain3/1 -> Sum5/2
  Integrator1/1 -> Gain3/1, at c/1

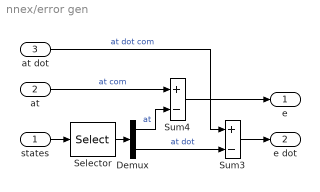
== system nnex/error gen ==
  states : Inport  Port=1  PortWidth=-1  SampleTime=-1  DataType=auto
      settings: SignalType=auto
  at : Inport  Port=2  PortWidth=-1  SampleTime=-1  DataType=auto
      settings: SignalType=auto
  at dot : Inport  Port=3  PortWidth=-1  SampleTime=-1  DataType=auto
      settings: SignalType=auto
  Demux : Demux  Outputs=2
  Selector : Selector  Elements=[1 2 3 7 8 9]  InputPortWidth=9
  Sum3 : Sum  Inputs=+-  SaturateOnIntegerOverflow=on
  Sum4 : Sum  Inputs=+-  SaturateOnIntegerOverflow=on
  e : Outport  Port=1
  e dot : Outport  Port=2
  wires:
  Sum3/1 -> e dot/1
  Sum4/1 -> e/1
  Demux/2 -> Sum3/2  "at dot"
  Demux/1 -> Sum4/2  "at"
  at/1 -> Sum4/1  "at com"
  at dot/1 -> Sum3/1  "at dot com"
  Selector/1 -> Demux/1
  states/1 -> Selector/1
